simulink model "sf_while"  (Simulink 7.6)
settings: Solver=FixedStepDiscrete  StartTime=0.0  StopTime=1  FixedStep=1  RelTol=1e-3
settings Model: Creator=The MathWorks Inc.  CovMetricSettings=dcmtr  ExtModeAutoUpdateStatusClock=off
settings DataIOCC: SignalLoggingName=sigsOut
settings OptimizationCC: InlineInvariantSignals=on  InitFltsAndDblsToZero=on  EfficientMapNaN2IntZero=off
settings DebuggingCC: SaveWithParameterizedLinksMsg=none  SignalResolutionControl=TryResolveAllWithWarning  SolverPrmCheckMsg=none  MultiTaskDSMMsg=warning  MultiTaskCondExecSysMsg=none  StrictBusMsg=None
settings HardwareCC: TargetUnknown=on
settings SFSimCC: SimParseCustomCode=off
settings RTWCC: IncludeERTFirstTime=on
settings GRTTargetCC: TargetFcnLib=ansi_tfl_tmw.mat

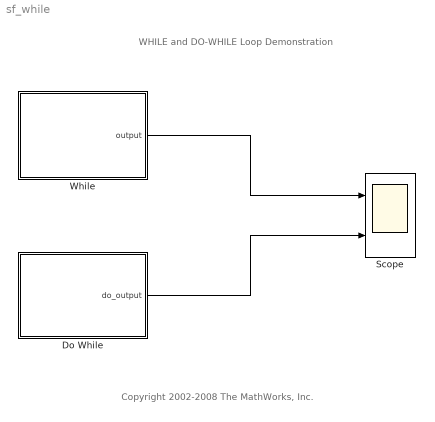
== system sf_while ==
  note: WHILE and DO-WHILE Loop Demonstration
  note: Copyright 2002-2008 The MathWorks, Inc.
  Do While : Stateflow chart  TreatAsAtomicUnit=on
  Scope : Scope  NumInputPorts=2
      settings: TimeRange=1  YMin=0~0  YMax=20~20
  While : Stateflow chart  TreatAsAtomicUnit=on
  wires:
  Do While/1(do_output) -> Scope/2
  While/1(output) -> Scope/1

== stateflow chart While ==
  note: Equivalent C-Code:
      |
      | while(condition < 20)
      | {
      |     while_output[i] = condition;
      |     i++;
      |     condition+=2;
      | }
  (default) -> (junction 4)
  (junction 5) -> (junction 4) [order 1] : [condition < 20]
      | {while_output[i] =condition;i++;
      | condition+=2;}
  (junction 4) -> (junction 5)
  (junction 5) -> (junction 6) [order 2] : {output=while_output;}
  data: condition local double; output output double size=[10 1]; i local double; while_output local double size=[10 1]

== stateflow chart Do While ==
  note: Equivalent C-Code
      |
      | do {
      |       do_output[i]=condition;
      |       condition+=2;
      |       i++;
      |      } while(condition<20);
  (default) -> (junction 18)
  (junction 18) -> (junction 19) : {do_output[i]=condition;}
  (junction 19) -> (junction 20) [order 2] : {do_output;}
  (junction 19) -> (junction 18) [order 1] : [condition<20]{condition+=2;i++;}
  data: i local double; do_output output double size=[11]; condition local double
